simulink model "F303RE_I2S_Test"  (R2018b)
settings: Solver=FixedStepDiscrete  StartTime=0.0  StopTime=10.0  FixedStep=0.01  RelTol=1e-3
libraries: I2S_Lib x11, GPIO_Lib x7, SPI_Lib x2, DAC_Lib x1, STM32_Config_Lib x1, TIMERS_Lib x1
settings Model: Creator=reynaudp  LastModifiedBy=fenard1
settings DataIOCC: ReturnWorkspaceOutputs=on
settings OptimizationCC: DefaultParameterBehavior=Inlined  DefaultUnderspecifiedDataType=single
settings DebuggingCC: ReadBeforeWriteMsg=DisableAll  WriteAfterWriteMsg=DisableAll  WriteAfterReadMsg=DisableAll  MultiTaskDSMMsg=none  ParameterTunabilityLossMsg=error  SFUndirectedBroadcastEventsDiag=error
settings HardwareCC: ProdBitPerPointer=32  ProdBitPerSizeT=32  ProdBitPerPtrDiffT=32  ProdLargestAtomicInteger=Integer  ProdWordSize=32  ProdHWDeviceType=STMicroelectronics->STM32 32-bit Cortex-M
settings ModelReferenceCC: UpdateModelReferenceTargets=IfOutOfDate
settings SFSimCC: SFSimEcho=off  SimUseLocalCustomCode=off  CompileTimeRecursionLimit=0  EnableRuntimeRecursion=off  MATLABDynamicMemAlloc=off
settings RTWCC: SystemTargetFile=stm32.tlc  TemplateMakefile=stm32.tmf  Description=stm32 (Embedded Target)  GenerateReport=on  RTWUseLocalCustomCode=off  IncludeHyperlinkInReport=on
settings CodeAppCC: ForceParamTrailComments=on  IgnoreCustomStorageClasses=off  OperatorAnnotations=on  SimulinkDataObjDesc=on  SFDataObjDesc=on  MATLABFcnDesc=on  CustomSymbolStrType=$N$R$M  SimulinkBlockComments=off  MATLABSourceComments=on
settings STFCustomTargetCC: TargetLangStandard=C99 (ISO)  ParMdlRefBuildCompliant=on  IncludeMdlTerminateFcn=off  CombineOutputUpdateFcns=on  ERTCustomFileBanners=on  SupportNonFinite=off  SupportComplex=off  SupportContinuousTime=off  SupportNonInlinedSFcns=off  RemoveResetFunc=on  ParenthesesLevel=Maximum  CastingMode=Standards  MATLABClassNameForMDSCustomization=Simulink.SoftwareTarget.ERTCustomization  SystemTargetFile=stm32.tlc
settings ERTTargetCC: TargetLangStandard=C99 (ISO)  MultiwordLength=2048  CompOptLevelCompliant=off  ConcurrentExecutionCompliant=off  IncludeMdlTerminateFcn=off  SupportNonFinite=off  SupportComplex=off  ParenthesesLevel=Maximum  CastingMode=Standards  ModelStepFunctionPrototypeControlCompliant=off  CPPClassGenCompliant=off  UseToolchainInfoCompliant=off  ExtModeStaticAllocSize=256  ExtModeMexArgs=0,1,115200,10  InlinedParameterPlacement=NonHierarchical  ERTSrcFileBannerTemplate=sourceFileTemplate.cgt  ERTHdrFileBannerTemplate=sourceFileTemplate.cgt  ERTDataSrcFileTemplate=sourceFileTemplate.cgt  ERTDataHdrFileTemplate=sourceFileTemplate.cgt  ERTCustomFileTemplate=customRoutineProcess.tlc  PreserveIfCondition=on  EnableSignedLeftShifts=off  EnableSignedRightShifts=off

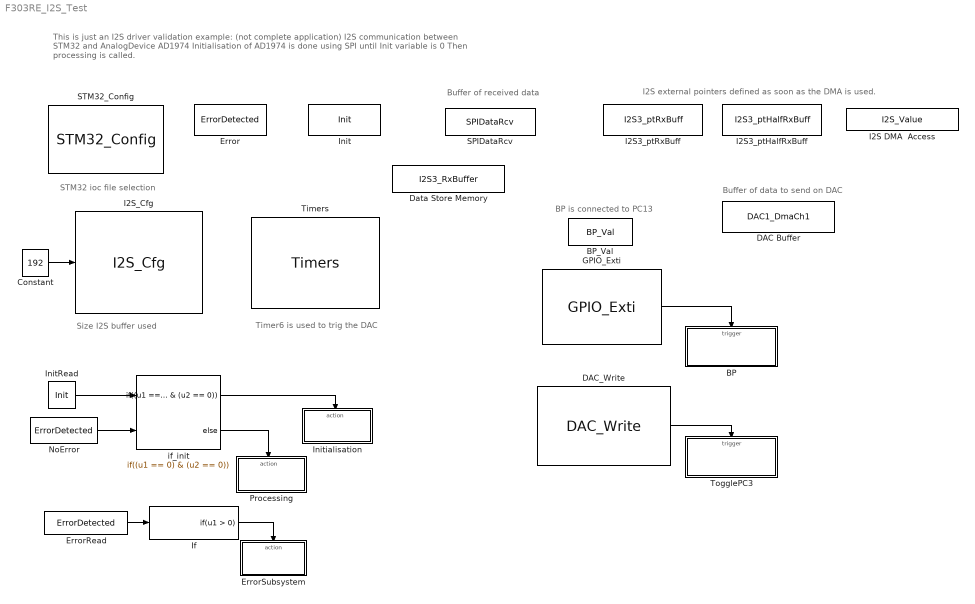
== system F303RE_I2S_Test ==
  note: Size I2S buffer used
  note: Timer6 is used to trig the DAC
  note: BP is connected to PC13
  note: Buffer of data to send on DAC
  note: Buffer of received data
  note: I2S external pointers defined as soon as the DMA is used.
  note: This is just an I2S driver validation example: (not complete application)
      | I2S communication between STM32 and AnalogDevice AD1974
      | Initialisation of AD1974 is done using SPI until Init variable is 0
      | Then processing is called.
  note: STM32 ioc file selection
  BP : Subsystem  TreatAsAtomicUnit=on
  BP_Val : DataStoreMemory  DataStoreName=BP_Val  ReadBeforeWriteMsg=warning  WriteAfterWriteMsg=warning  WriteAfterReadMsg=warning  InitialValue=1  ShowAdditionalParam=off  OutDataTypeStr=uint8
  Constant : Constant  Value=192  OutDataTypeStr=uint8
  DAC Buffer : DataStoreMemory  DataStoreName=DAC1_DmaCh1  ReadBeforeWriteMsg=warning  WriteAfterWriteMsg=warning  WriteAfterReadMsg=warning  ShowAdditionalParam=off  OutDataTypeStr=uint16  Dimensions=48
      settings: RTWStateStorageClass=ImportedExternPointer
  DAC_Write : DAC_Lib/DAC_Write  DAC_Name=DAC1  Pin0=off  Pin1=off  Align=12bit_right  DmaBuffCh1=48  DmaBuffCh2=0  CpltTrans=on  HalfTrans=off  ErrorIt=off  UnderIt=off  NbDAC=1  UsedDma=on
      settings: SourceProductName=Target Support Package - STM32 Adapter
  Data Store Memory : DataStoreMemory  DataStoreName=I2S3_RxBuffer  ReadBeforeWriteMsg=warning  WriteAfterWriteMsg=warning  WriteAfterReadMsg=warning  ShowAdditionalParam=off  Dimensions=192
  Error : DataStoreMemory  DataStoreName=ErrorDetected  ReadBeforeWriteMsg=warning  WriteAfterWriteMsg=warning  WriteAfterReadMsg=warning  ShowAdditionalParam=off  OutDataTypeStr=uint8
  ErrorRead : DataStoreRead  DataStoreName=ErrorDetected
  ErrorSubsystem : Subsystem  TreatAsAtomicUnit=on
  GPIO_Exti : GPIO_Lib/GPIO_Exti  Port_name=GPIOC  Pin_0=off  Pin_1=off  Pin_2=off  Pin_3=off  Pin_4=off  Pin_5=off  Pin_6=off  Pin_7=off  Pin_8=off  Pin_9=off  Pin_10=off  Pin_11=off  Pin_12=off  Pin_13=on  Pin_14=off  Pin_15=off  PinList=GPIOA9GPIOC13
      settings: SourceProductName=Target Support Package - STM32 Adapter
  I2S DMA  Access : DataStoreMemory  DataStoreName=I2S_Value  ReadBeforeWriteMsg=warning  WriteAfterWriteMsg=warning  WriteAfterReadMsg=warning  ShowAdditionalParam=off  OutDataTypeStr=uint16  Dimensions=96
  I2S3_ptHalfRxBuff : DataStoreMemory  DataStoreName=I2S3_ptHalfRxBuff  ReadBeforeWriteMsg=warning  WriteAfterWriteMsg=warning  WriteAfterReadMsg=warning  ShowAdditionalParam=off  OutDataTypeStr=uint16  Dimensions=96
      settings: RTWStateStorageClass=ImportedExternPointer
  I2S3_ptRxBuff : DataStoreMemory  DataStoreName=I2S3_ptRxBuff  ReadBeforeWriteMsg=warning  WriteAfterWriteMsg=warning  WriteAfterReadMsg=warning  ShowAdditionalParam=off  OutDataTypeStr=uint16  Dimensions=96
      settings: RTWStateStorageClass=ImportedExternPointer
  I2S_Cfg : I2S_Lib/I2S_Cfg  I2Sx=I2S3  Master_Slave=MASTER  Half_Full=HALF DUPLEX  Rx_Tx=Receiver  I2S_Mode=DMA_RX  NbI2S=1  Rx_SizeIn=off  Rx_Size=192  Tx_SizeIn=on  Tx_Size=192
      settings: SourceProductName=Target Support Package - STM32 Adapter  DataFormat=16 Bits Data on 32 Bits Frame
  If : If  ShowElse=off
  Init : DataStoreMemory  DataStoreName=Init  ReadBeforeWriteMsg=warning  WriteAfterWriteMsg=warning  WriteAfterReadMsg=warning  ShowAdditionalParam=off  OutDataTypeStr=uint8
  InitRead : DataStoreRead  DataStoreName=Init
  Initialisation : Subsystem  TreatAsAtomicUnit=on
  NoError : DataStoreRead  DataStoreName=ErrorDetected
  Processing : Subsystem  TreatAsAtomicUnit=on
  SPIDataRcv : DataStoreMemory  DataStoreName=SPIDataRcv  ReadBeforeWriteMsg=warning  WriteAfterWriteMsg=warning  WriteAfterReadMsg=warning  ShowAdditionalParam=off  OutDataTypeStr=uint8  Dimensions=3
  STM32_Config : STM32_Config_Lib/STM32_Config  Priority=0  Project_Path=.\  Config_File=F303RE.ioc  MCU_Name=STM32F303RETx
      settings: SourceProductName=Target Support Package - STM32 Adapter
  Timers : TIMERS_Lib/Timers  currentTIM=TIM6  TIM_Name=TIM6  sysUsingTimer=on  TIM_APBClock=72000000  TIM_Set_Clk=off  TIM_Prescaler=9  TIM_Clock=7200000.00  Variable_frequency=off  TIM_Set_OutFreq=on  TIM_ARR=150  Output_frequency=48000.00  Repetition_counter=0  TIM_Mode=Up  TIM_DMA=none  TIM_IRQ=off  TIM_IRQ_ONLY=on  TIM_UP=off  TIM_TRG=off  TIM_COM=off  TIM_BRK=off  NbTIM=1  CH1_enable=off  CH1N_enable=off  CH1_type=Unknown  CH1_DMA=off  CH1_int=off  CH1_edge=Rising  CH1_div=1  CH1_variable_duty=off  CH1_set_pulse=off  CH1_output_duty=0.00  CH1_pulse=0  CH2_enable=off  CH2N_enable=off  CH2_type=Unknown  CH2_DMA=off  CH2_int=off  CH2_edge=Rising  CH2_div=1  CH2_variable_duty=off  CH2_set_pulse=off  CH2_output_duty=0.00  CH2_pulse=0  CH3_enable=off  CH3N_enable=off  CH3_type=Unknown  CH3_DMA=off  CH3_int=off  CH3_edge=Rising  CH3_div=1  CH3_variable_duty=off  CH3_set_pulse=off  CH3_output_duty=0.00  CH3_pulse=0  CH4_enable=off  CH4N_enable=off  CH4_type=Unknown  CH4_DMA=off  CH4_int=off  CH4_edge=Rising  CH4_div=1  CH4_variable_duty=off  CH4_set_pulse=off  CH4_output_duty=0.00  CH4_pulse=0
      settings: SourceProductName=Target Support Package - STM32 Adapter
  TogglePC3 : Subsystem  TreatAsAtomicUnit=on
  if_init : If  NumInputs=2  IfExpression=(u1 == 0) & (u2 == 0)
  wires:
  ErrorRead/1 -> If/1
  If/1 -> ErrorSubsystem/Action
  InitRead/1 -> if_init/1
  NoError/1 -> if_init/2
  if_init/1 -> Initialisation/Action
  if_init/2 -> Processing/Action
  DAC_Write/1 -> TogglePC3/Trigger
  GPIO_Exti/1 -> BP/Trigger
  Constant/1 -> I2S_Cfg/1

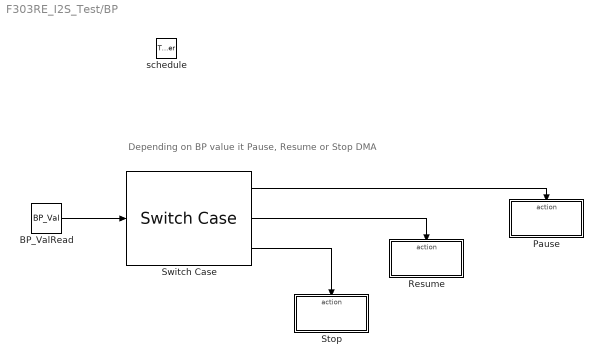
== system F303RE_I2S_Test/BP ==
  note: Depending on BP value it Pause, Resume or Stop DMA
  schedule : TriggerPort  TriggerType=function-call  VariantControl=Variant
  BP_ValRead : DataStoreRead  DataStoreName=BP_Val
  Pause : Subsystem  TreatAsAtomicUnit=on
  Resume : Subsystem  TreatAsAtomicUnit=on
  Stop : Subsystem  TreatAsAtomicUnit=on
  Switch Case : SwitchCase  CaseConditions={1,2,3}  ShowDefaultCase=off
  wires:
  BP_ValRead/1 -> Switch Case/1
  Switch Case/1 -> Pause/Action
  Switch Case/2 -> Resume/Action
  Switch Case/3 -> Stop/Action

== system F303RE_I2S_Test/ErrorSubsystem ==
  note: Blink LED
  Action Port : ActionPort  ActionType=then
  GPIO_Write : GPIO_Lib/GPIO_Write  Port_name=GPIOB  Pin0=off  Toggle_Pin0=off  Pin1=off  Toggle_Pin1=off  Pin2=off  Toggle_Pin2=off  Pin3=off  Toggle_Pin3=off  Pin4=off  Toggle_Pin4=off  Pin5=off  Toggle_Pin5=off  Pin6=off  Toggle_Pin6=off  Pin7=off  Toggle_Pin7=off  Pin8=off  Toggle_Pin8=off  Pin9=off  Toggle_Pin9=off  Pin10=off  Toggle_Pin10=off  Pin11=off  Toggle_Pin11=off  Pin12=off  Toggle_Pin12=off  Pin13=off  Toggle_Pin13=off  Pin14=off  Toggle_Pin14=off  Pin15=off  Toggle_Pin15=off  PinList="GPIOA8  10GPIOB3  6GPIOC3"
      settings: SourceProductName=Target Support Package - STM32 Adapter

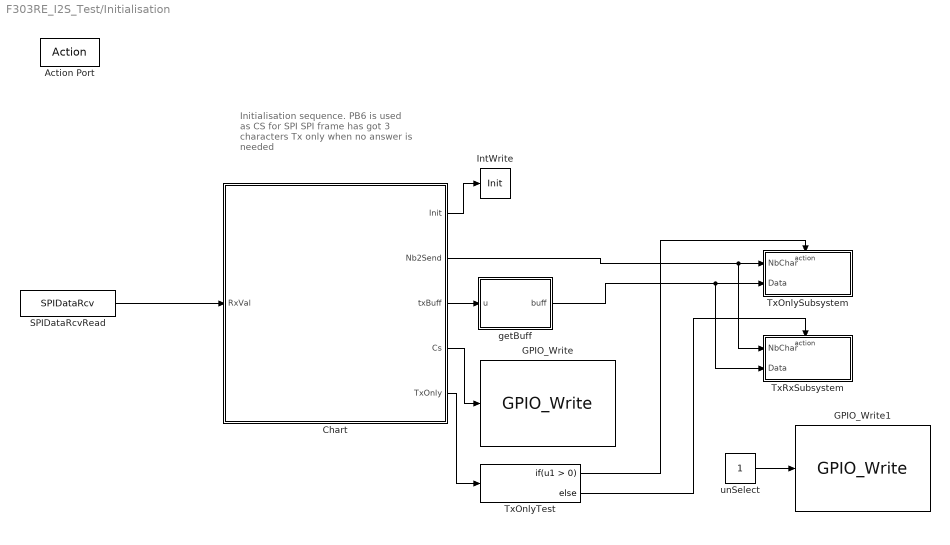
== system F303RE_I2S_Test/Initialisation ==
  note: Initialisation sequence.
      | PB6 is used as CS for SPI
      | SPI frame has got 3 characters
      | Tx only when no answer is needed
  Action Port : ActionPort  ActionType=then
  Chart : Stateflow chart  TreatAsAtomicUnit=on
  GPIO_Write : GPIO_Lib/GPIO_Write  Priority=0  Port_name=GPIOB  Pin0=off  Toggle_Pin0=off  Pin1=off  Toggle_Pin1=off  Pin2=off  Toggle_Pin2=off  Pin3=off  Toggle_Pin3=off  Pin4=off  Toggle_Pin4=off  Pin5=off  Toggle_Pin5=off  Pin6=on  Toggle_Pin6=off  Pin7=off  Toggle_Pin7=off  Pin8=off  Toggle_Pin8=off  Pin9=off  Toggle_Pin9=off  Pin10=off  Toggle_Pin10=off  Pin11=off  Toggle_Pin11=off  Pin12=off  Toggle_Pin12=off  Pin13=off  Toggle_Pin13=off  Pin14=off  Toggle_Pin14=off  Pin15=off  Toggle_Pin15=off  PinList="GPIOA8  10GPIOB3  6GPIOC3"
      settings: SourceProductName=Target Support Package - STM32 Adapter
  GPIO_Write1 : GPIO_Lib/GPIO_Write  Priority=2  Port_name=GPIOB  Pin0=off  Toggle_Pin0=off  Pin1=off  Toggle_Pin1=off  Pin2=off  Toggle_Pin2=off  Pin3=off  Toggle_Pin3=off  Pin4=off  Toggle_Pin4=off  Pin5=off  Toggle_Pin5=off  Pin6=on  Toggle_Pin6=off  Pin7=off  Toggle_Pin7=off  Pin8=off  Toggle_Pin8=off  Pin9=off  Toggle_Pin9=off  Pin10=off  Toggle_Pin10=off  Pin11=off  Toggle_Pin11=off  Pin12=off  Toggle_Pin12=off  Pin13=off  Toggle_Pin13=off  Pin14=off  Toggle_Pin14=off  Pin15=off  Toggle_Pin15=off  PinList="GPIOA8  10GPIOB3  6GPIOC3"
      settings: SourceProductName=Target Support Package - STM32 Adapter
  IntWrite : DataStoreWrite  DataStoreName=Init
  SPIDataRcvRead : DataStoreRead  DataStoreName=SPIDataRcv
  TxOnlySubsystem : Subsystem  TreatAsAtomicUnit=on
  TxOnlyTest : If
  TxRxSubsystem : Subsystem  TreatAsAtomicUnit=on
  getBuff : MATLAB Function  TreatAsAtomicUnit=on
  unSelect : Constant
  wires:
  Chart/1(Init) -> IntWrite/1
  Chart/3(txBuff) -> getBuff/1(u)
  Chart/4(Cs) -> GPIO_Write/1
  unSelect/1 -> GPIO_Write1/1
  Chart/5(TxOnly) -> TxOnlyTest/1
  TxOnlyTest/1 -> TxOnlySubsystem/Action
  TxOnlyTest/2 -> TxRxSubsystem/Action
  Chart/2(Nb2Send) -> TxRxSubsystem/1(NbChar), TxOnlySubsystem/1(NbChar)
  getBuff/1(buff) -> TxRxSubsystem/2(Data), TxOnlySubsystem/2(Data)
  SPIDataRcvRead/1 -> Chart/1(RxVal)

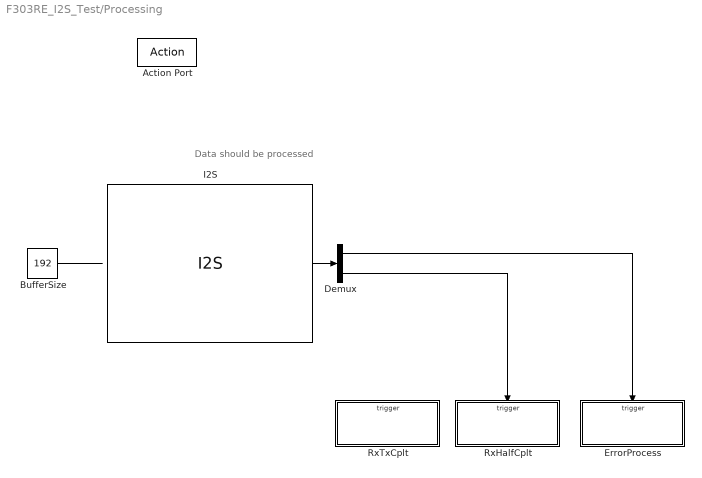
== system F303RE_I2S_Test/Processing ==
  note: Data should be processed
  Action Port : ActionPort  ActionType=else
  BufferSize : Constant  Value=192
  Demux : Demux  Outputs=2
  ErrorProcess : Subsystem  TreatAsAtomicUnit=on
  I2S : I2S_Lib/I2S  I2Sx=I2S3  Master_Slave=MASTER  Half_Full=HALF DUPLEX  Rx_Tx=Receiver  ptDataSent=off  Protocol=I2S Philips  Frequency=48 KHz  RealFrequency=46.875 KHz  FrequencyError=-2.34 %  ClockPol=Low  I2S_Mode=DMA_RX  Timeout=-1  TimeoutValue=0.01  handler=hi2s3  NbI2S=1  Error=on  RxHalfCplt=on  RxCplt=off  TxHalfCplt=off  TxCplt=off  RxTxCplt=off  outputData=off
      settings: SourceProductName=Target Support Package - STM32 Adapter  DataFormat=16 Bits Data on 32 Bits Frame
  RxHalfCplt : Subsystem  TreatAsAtomicUnit=on
  RxTxCplt : Subsystem  TreatAsAtomicUnit=on
  wires:
  BufferSize/1 -> ?
  I2S/1 -> Demux/1
  Demux/1 -> ErrorProcess/Trigger
  Demux/2 -> RxHalfCplt/Trigger

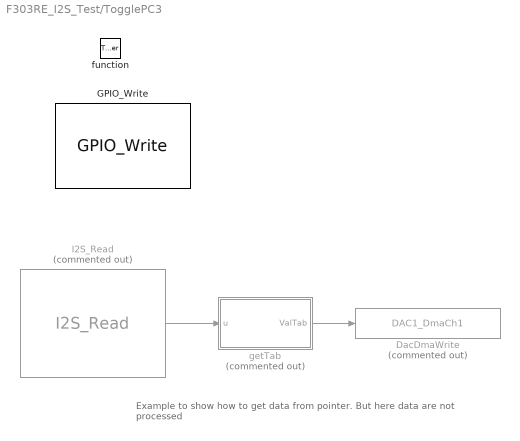
== system F303RE_I2S_Test/TogglePC3 ==
  note: Example to show how to get data from pointer.
      |
      | But here data are not processed
  function : TriggerPort  TriggerType=function-call  VariantControl=Variant
  DacDmaWrite : DataStoreWrite  Commented=on  DataStoreName=DAC1_DmaCh1
  GPIO_Write : GPIO_Lib/GPIO_Write  Port_name=GPIOB  Pin0=off  Toggle_Pin0=off  Pin1=off  Toggle_Pin1=off  Pin2=off  Toggle_Pin2=off  Pin3=off  Toggle_Pin3=off  Pin4=off  Toggle_Pin4=off  Pin5=off  Toggle_Pin5=off  Pin6=off  Toggle_Pin6=off  Pin7=off  Toggle_Pin7=off  Pin8=off  Toggle_Pin8=off  Pin9=off  Toggle_Pin9=off  Pin10=off  Toggle_Pin10=off  Pin11=off  Toggle_Pin11=off  Pin12=off  Toggle_Pin12=off  Pin13=off  Toggle_Pin13=off  Pin14=off  Toggle_Pin14=off  Pin15=off  Toggle_Pin15=off  PinList="GPIOA8  10GPIOB3  6GPIOC3"
      settings: SourceProductName=Target Support Package - STM32 Adapter
  I2S_Read : I2S_Lib/I2S_Read  Commented=on  I2Sx=I2S3  OffsetIn=off  OffsetVal=0  outputData=on
      settings: SourceProductName=Target Support Package - STM32 Adapter
  getTab : MATLAB Function  Commented=on  TreatAsAtomicUnit=on
  wires:
  I2S_Read/2 -> getTab/1(u)
  getTab/1(ValTab) -> DacDmaWrite/1

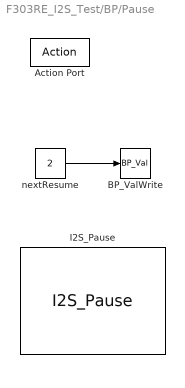
== system F303RE_I2S_Test/BP/Pause ==
  Action Port : ActionPort  ActionType=case
  BP_ValWrite : DataStoreWrite  DataStoreName=BP_Val
  I2S_Pause : I2S_Lib/I2S_Pause  I2Sx=I2S3
      settings: SourceProductName=Target Support Package - STM32 Adapter
  nextResume : Constant  Value=2  OutDataTypeStr=uint8
  wires:
  nextResume/1 -> BP_ValWrite/1

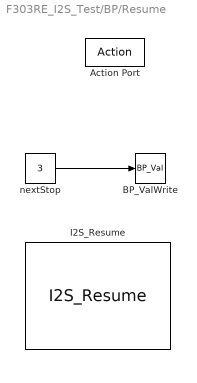
== system F303RE_I2S_Test/BP/Resume ==
  Action Port : ActionPort  ActionType=case
  BP_ValWrite : DataStoreWrite  DataStoreName=BP_Val
  I2S_Resume : I2S_Lib/I2S_Resume  I2Sx=I2S3
      settings: SourceProductName=Target Support Package - STM32 Adapter
  "nextStop " : Constant  Value=3  OutDataTypeStr=uint8
  wires:
  "nextStop "/1 -> BP_ValWrite/1

== system F303RE_I2S_Test/BP/Stop ==
  Action Port : ActionPort  ActionType=case
  BP_ValWrite : DataStoreWrite  DataStoreName=BP_Val
  I2S_Stop : I2S_Lib/I2S_Stop  I2Sx=I2S3
      settings: SourceProductName=Target Support Package - STM32 Adapter
  nextEnd : Constant  Value=0  OutDataTypeStr=uint8
  wires:
  nextEnd/1 -> BP_ValWrite/1

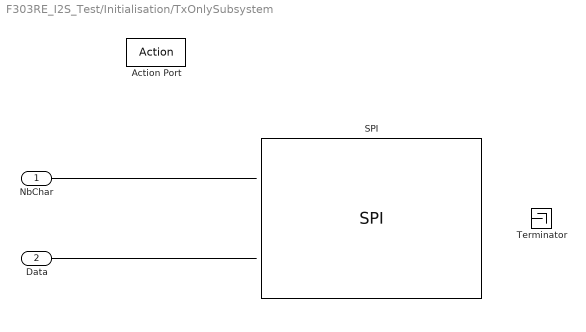
== system F303RE_I2S_Test/Initialisation/TxOnlySubsystem ==
  NbChar : Inport
  Data : Inport  Port=2
  Action Port : ActionPort  ActionType=then
  SPI : SPI_Lib/SPI  SPIx=SPI1  Device_Mode=MASTER  Type_SPI=Full_Duplex  SPI_Mode=POLLING  TxOnly=on  handler=hspi1  Buffer_Size_Rcv=32  Buffer_Size_Send=32  NbSPI=1  BaudRate=1.125 MBits/s  Nb_bits_transmission=8  Timeout=200  TimeoutValue=2  NSS=off  Error=off  CallBack=off  Transmission=off  outputData=off
      settings: SourceProductName=Target Support Package - STM32 Adapter
  Terminator : Terminator
  wires:
  NbChar/1 -> ?
  Data/1 -> ?
  ? -> Terminator/1

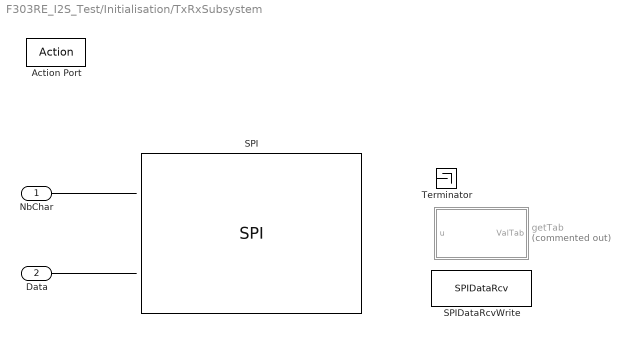
== system F303RE_I2S_Test/Initialisation/TxRxSubsystem ==
  NbChar : Inport
  Data : Inport  Port=2
  Action Port : ActionPort  ActionType=else
  SPI : SPI_Lib/SPI  Priority=1  SPIx=SPI1  Device_Mode=MASTER  Type_SPI=Full_Duplex  SPI_Mode=POLLING  TxOnly=off  handler=hspi1  Buffer_Size_Rcv=3  Buffer_Size_Send=3  NbSPI=1  BaudRate=1.125 MBits/s  Nb_bits_transmission=8  Timeout=200  TimeoutValue=2  NSS=off  Error=off  CallBack=off  Transmission=off  outputData=on
      settings: SourceProductName=Target Support Package - STM32 Adapter
  SPIDataRcvWrite : DataStoreWrite  DataStoreName=SPIDataRcv
  Terminator : Terminator
  getTab : MATLAB Function  Commented=on  TreatAsAtomicUnit=on
  wires:
  NbChar/1 -> ?
  Data/1 -> ?
  ? -> SPIDataRcvWrite/1
  ? -> getTab/1(u)
  ? -> Terminator/1

== system F303RE_I2S_Test/Processing/ErrorProcess ==
  ProcessError : TriggerPort  TriggerType=function-call  VariantControl=Variant
  Constant : Constant  OutDataTypeStr=uint8
  ErrorWrite : DataStoreWrite  DataStoreName=ErrorDetected
  wires:
  Constant/1 -> ErrorWrite/1

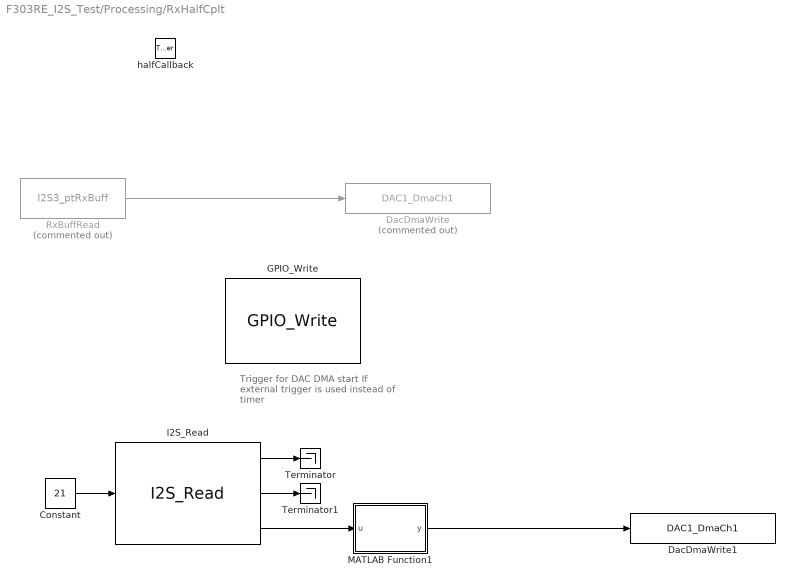
== system F303RE_I2S_Test/Processing/RxHalfCplt ==
  note: Trigger for DAC DMA start
      | If external trigger is used instead of timer
  halfCallback : TriggerPort  TriggerType=function-call  VariantControl=Variant
  Constant : Constant  Value=21  OutDataTypeStr=uint16
  DacDmaWrite : DataStoreWrite  Commented=on  DataStoreName=DAC1_DmaCh1
  DacDmaWrite1 : DataStoreWrite  DataStoreName=DAC1_DmaCh1
  GPIO_Write : GPIO_Lib/GPIO_Write  Port_name=GPIOB  Pin0=off  Toggle_Pin0=off  Pin1=off  Toggle_Pin1=off  Pin2=off  Toggle_Pin2=off  Pin3=off  Toggle_Pin3=off  Pin4=off  Toggle_Pin4=off  Pin5=off  Toggle_Pin5=off  Pin6=off  Toggle_Pin6=off  Pin7=off  Toggle_Pin7=off  Pin8=off  Toggle_Pin8=off  Pin9=off  Toggle_Pin9=off  Pin10=off  Toggle_Pin10=off  Pin11=off  Toggle_Pin11=off  Pin12=off  Toggle_Pin12=off  Pin13=off  Toggle_Pin13=off  Pin14=off  Toggle_Pin14=off  Pin15=off  Toggle_Pin15=off  PinList="GPIOA8  10GPIOB3  6GPIOC3"
      settings: SourceProductName=Target Support Package - STM32 Adapter
  I2S_Read : I2S_Lib/I2S_Read  I2Sx=I2S3  OffsetIn=on  OffsetVal=0  outputData=on
      settings: SourceProductName=Target Support Package - STM32 Adapter
  MATLAB Function1 : MATLAB Function  TreatAsAtomicUnit=on
  RxBuffRead : DataStoreRead  Commented=on  DataStoreName=I2S3_ptRxBuff
  Terminator : Terminator
  Terminator1 : Terminator
  wires:
  RxBuffRead/1 -> DacDmaWrite/1
  I2S_Read/3 -> MATLAB Function1/1(u)
  MATLAB Function1/1(y) -> DacDmaWrite1/1
  Constant/1 -> I2S_Read/1
  I2S_Read/1 -> Terminator/1
  I2S_Read/2 -> Terminator1/1

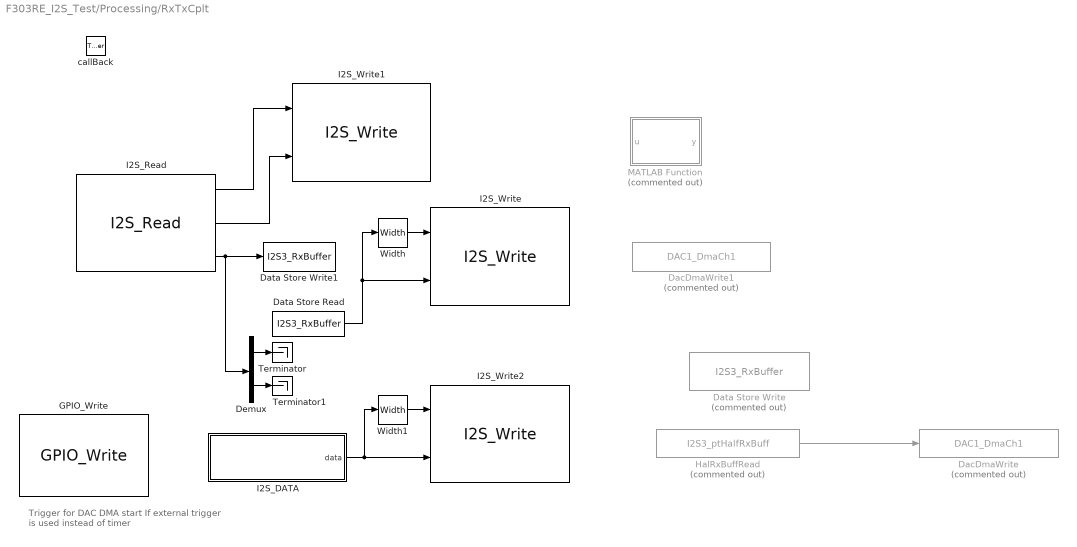
== system F303RE_I2S_Test/Processing/RxTxCplt ==
  note: Trigger for DAC DMA start
      | If external trigger is used instead of timer
  callBack : TriggerPort  TriggerType=function-call  VariantControl=Variant
  DacDmaWrite : DataStoreWrite  Commented=on  DataStoreName=DAC1_DmaCh1
  DacDmaWrite1 : DataStoreWrite  Commented=on  DataStoreName=DAC1_DmaCh1
  Data Store Read : DataStoreRead  DataStoreName=I2S3_RxBuffer
  Data Store Write : DataStoreWrite  Commented=on  DataStoreName=I2S3_RxBuffer
  Data Store Write1 : DataStoreWrite  DataStoreName=I2S3_RxBuffer
  Demux : Demux  Outputs=2
  GPIO_Write : GPIO_Lib/GPIO_Write  Port_name=GPIOB  Pin0=off  Toggle_Pin0=off  Pin1=off  Toggle_Pin1=off  Pin2=off  Toggle_Pin2=off  Pin3=off  Toggle_Pin3=off  Pin4=off  Toggle_Pin4=off  Pin5=off  Toggle_Pin5=off  Pin6=off  Toggle_Pin6=off  Pin7=off  Toggle_Pin7=off  Pin8=off  Toggle_Pin8=off  Pin9=off  Toggle_Pin9=off  Pin10=off  Toggle_Pin10=off  Pin11=off  Toggle_Pin11=off  Pin12=off  Toggle_Pin12=off  Pin13=off  Toggle_Pin13=off  Pin14=off  Toggle_Pin14=off  Pin15=off  Toggle_Pin15=off  PinList="GPIOA8  10GPIOB3  6GPIOC3"
      settings: SourceProductName=Target Support Package - STM32 Adapter
  HalRxBuffRead : DataStoreRead  Commented=on  DataStoreName=I2S3_ptHalfRxBuff
  I2S_DATA : Subsystem
  I2S_Read : I2S_Lib/I2S_Read  I2Sx=I2S3  OffsetIn=off  OffsetVal=3  outputData=on
      settings: SourceProductName=Target Support Package - STM32 Adapter
  I2S_Write : I2S_Lib/I2S_Write  I2Sx=I2S3  inputData=on  dataMsg=BufferDataSend is the data to copy to the send buffer  OffsetIn=off  OffsetVal=12
      settings: SourceProductName=Target Support Package - STM32 Adapter  DataFormat=16 Bits Data on 32 Bits Frame
  I2S_Write1 : I2S_Lib/I2S_Write  I2Sx=I2S3  inputData=off  dataMsg=ptDataSend is the address of the data to copy to the send buffer  OffsetIn=off  OffsetVal=50
      settings: SourceProductName=Target Support Package - STM32 Adapter  DataFormat=16 Bits Data on 32 Bits Frame
  I2S_Write2 : I2S_Lib/I2S_Write  I2Sx=I2S3  inputData=on  dataMsg=BufferDataSend is the data to copy to the send buffer  OffsetIn=off  OffsetVal=12
      settings: SourceProductName=Target Support Package - STM32 Adapter  DataFormat=16 Bits Data on 32 Bits Frame
  MATLAB Function : MATLAB Function  Commented=on  TreatAsAtomicUnit=on
  Terminator : Terminator
  Terminator1 : Terminator
  Width : Width
  Width1 : Width
  wires:
  HalRxBuffRead/1 -> DacDmaWrite/1
  I2S_Read/3 -> Demux/1, Data Store Write1/1
  I2S_Read/1 -> I2S_Write1/1
  I2S_Read/2 -> I2S_Write1/2
  Data Store Read/1 -> Width/1, I2S_Write/2
  Width/1 -> I2S_Write/1
  I2S_DATA/1(data) -> Width1/1, I2S_Write2/2
  Width1/1 -> I2S_Write2/1
  Demux/1 -> Terminator/1
  Demux/2 -> Terminator1/1

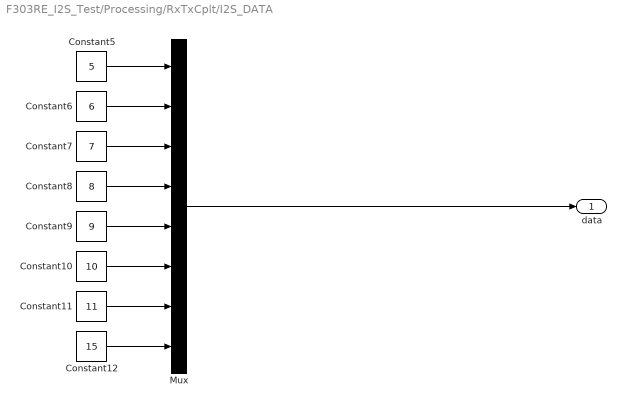
== system F303RE_I2S_Test/Processing/RxTxCplt/I2S_DATA ==
  Constant10 : Constant  Value=10  OutDataTypeStr=uint8
  Constant11 : Constant  Value=11  OutDataTypeStr=uint8
  Constant12 : Constant  Value=15  OutDataTypeStr=uint8
  Constant5 : Constant  Value=5  OutDataTypeStr=uint8
  Constant6 : Constant  Value=6  OutDataTypeStr=uint8
  Constant7 : Constant  Value=7  OutDataTypeStr=uint8
  Constant8 : Constant  Value=8  OutDataTypeStr=uint8
  Constant9 : Constant  Value=9  OutDataTypeStr=uint8
  Mux : Mux  Inputs=8
  data : Outport
  wires:
  Mux/1 -> data/1
  Constant5/1 -> Mux/1
  Constant6/1 -> Mux/2
  Constant9/1 -> Mux/5
  Constant10/1 -> Mux/6
  Constant7/1 -> Mux/3
  Constant12/1 -> Mux/8
  Constant8/1 -> Mux/4
  Constant11/1 -> Mux/7

== matlab function F303RE_I2S_Test/Initialisation/getBuff ==
  data: u input; buff output uint32 size=1
function buff = getBuff(u)
if coder.target('Sfun')
    % Executing in MATLAB, Buff is null
    buff = uint32(0);
else
    coder.cinclude('getBuffPtr.h');
    % Executing in the generated code.
    %buffer = zeros(1,3,'uint8');
    %coder.ceval('memcpy',coder.wref(buffer),coder.rref(u),3);
    %y = uint8(buffer(1:3));
    %buff = uint32(coder.ref(y));
    buff = coder.ceval('getBuffPtr',coder.rref(u));
end
end

== matlab function F303RE_I2S_Test/TogglePC3/getTab ==
  data: u input; ValTab output
function ValTab = I2SToDAC(u)
if coder.target('Sfun')
% Executing in MATLAB, Buff is null
ValTab = zeros(1,48,'uint8');
else
% Executing in the generated code. 
% Twist coder functions in order  to use input as a pointer.
ValTab = zeros(1,48,'uint8');
ptI2SData = coder.opaque('unsigned short*','0');
coder.ceval('ptI2SData=(unsigned short*)',u);
coder.ceval('memcpy',coder.wref(ValTab),ptI2SData,48);
end
end

== stateflow chart F303RE_I2S_Test/Initialisation/Chart ==
  state DumyRead
    en:
    txBuff[0] = uint8(9);
    txBuff[1] = uint8(0);
    txBuff[2] = uint8(0);
    ex: Nb2Send = uint8(3);
    Init = uint8(0);
    Cs = uint8(0);
    TxOnly = uint8(0);
  state DumyRead2
    entry: txBuff[0] = uint8(9);
    txBuff[1] = uint8(0);
    txBuff[2] = uint8(0);
    Nb2Send = uint8(3);
    Init = uint8(0);
    Cs = uint8(0);
    TxOnly = uint8(0);
  state DumyRead4
    entry: txBuff[0] = uint8(9);
    txBuff[1] = uint8(0);
    txBuff[2] = uint8(0);
    Nb2Send = uint8(3);
    Init = uint8(0);
    Cs = uint8(0);
    TxOnly = uint8(0);
  state WORDLENGTH_16
    entry: txBuff[0] = uint8(8);
    txBuff[1] = uint8(15);
    txBuff[2] = uint8(3);
    Nb2Send = uint8(3);
    Init = uint8(0);
    Cs = uint8(0);
    TxOnly = uint8(1);
  state PLL_OFF
    entry: txBuff[0] = uint8(8);
    txBuff[1] = uint8(0);
    txBuff[2] = uint8(1);
    Nb2Send = uint8(3);
    Init = uint8(0);
    Cs = uint8(0);
    TxOnly = uint8(1);
  state PLL_LOCK
    entry: txBuff[0] = uint8(9);
    txBuff[1] = uint8(1);
    txBuff[2] = uint8(0);
    Nb2Send = uint8(3);
    Init = uint8(0);
    Cs = uint8(0);
    TxOnly = uint8(0);
  state WORDLENGTH_Read
    entry: txBuff[0] = uint8(9);
    txBuff[1] = uint8(15);
    txBuff[2] = uint8(3);
    Nb2Send = uint8(3);
    Init = uint8(0);
    Cs = uint8(0);
    TxOnly = uint8(0);
  state DumyRead1
    entry: txBuff[0] = uint8(9);
    txBuff[1] = uint8(0);
    txBuff[2] = uint8(0);
    Nb2Send = uint8(3);
    Init = uint8(0);
    Cs = uint8(0);
    TxOnly = uint8(0);
  state HP_FILTER_ON
    entry: txBuff[0] = uint8(8);
    txBuff[1] = uint8(14);
    txBuff[2] = uint8(50);
    Nb2Send = uint8(3);
    Init = uint8(0);
    Cs = uint8(0);
    TxOnly = uint8(1);
  state ENABLE_PLL
    entry: txBuff[0] = uint8(8);
    txBuff[1] = uint8(0);
    txBuff[2] = uint8(72);
    Nb2Send = uint8(3);
    Init = uint8(0);
    Cs = uint8(0);
    TxOnly = uint8(1);
  state LRCK_IN
    entry: txBuff[0] = uint8(8);
    txBuff[1] = uint8(0);
    txBuff[2] = uint8(73);
    Nb2Send = uint8(3);
    Init = uint8(0);
    Cs = uint8(0);
    TxOnly = uint8(1);
  state DumyRead5
    entry: txBuff[0] = uint8(9);
    txBuff[1] = uint8(14);
    txBuff[2] = uint8(0);
    Nb2Send = uint8(3);
    Init = uint8(0);
    Cs = uint8(0);
    TxOnly = uint8(0);
  state START_CONERSION
    entry: txBuff[0] = uint16(8);
    txBuff[1] = uint16(0);
    txBuff[2] = uint16(200);
    Nb2Send = uint16(3);
    Init = uint8(0);
    Cs = uint8(0);
    TxOnly = uint8(1);
  state DumyRead6
    entry: txBuff[0] = uint16(9);
    txBuff[1] = uint16(0);
    txBuff[2] = uint16(0);
    Nb2Send = uint16(3);
    Init = uint8(1);
    Cs = uint8(0);
    TxOnly = uint8(0);
  (default) -> DumyRead
  LRCK_IN -> DumyRead2 : [1]
  ENABLE_PLL -> DumyRead4 : [1]
  DumyRead -> PLL_OFF : [after(0.5,sec)]
  DumyRead2 -> WORDLENGTH_16 : [RxVal[1] == 73||RxVal[2] == 73]
  DumyRead4 -> PLL_LOCK : [RxVal[1] == 72||RxVal[2] == 72]
  PLL_LOCK -> PLL_LOCK [order 1] : [RxVal[1] != 8&&RxVal[2] != 8 && after(0.5,sec)]
  WORDLENGTH_16 -> WORDLENGTH_Read : [1]
  PLL_OFF -> DumyRead1 : [1]
  PLL_LOCK -> HP_FILTER_ON [order 2] : [RxVal[1] == 8||RxVal[2] == 8]
  WORDLENGTH_Read -> ENABLE_PLL : [RxVal[1] == 3||RxVal[2] == 3]
  DumyRead1 -> LRCK_IN : [RxVal[1] == 1||RxVal[2] == 1]
  HP_FILTER_ON -> DumyRead5 : [1]
  DumyRead5 -> START_CONERSION : [RxVal[1] == 50||RxVal[2] == 50]
  START_CONERSION -> DumyRead6 : [1]
  data: Init output uint8; Nb2Send output uint16; RxVal input uint8 size=3; txBuff output uint8 size=3; Cs output uint8; TxOnly output uint8

== matlab function F303RE_I2S_Test/Initialisation/TxRxSubsystem/getTab ==
  data: u input; ValTab output
function ValTab = getElems(u)
if coder.target('Sfun')
% Executing in MATLAB, Buff is null
ValTab = zeros(1,3,'uint8');
else
% Executing in the generated code. 
% Twist coder functions in order  to use input as a pointer.
ValTab = zeros(1,3,'uint8');
pt2Data = coder.opaque('unsigned short*','0');
coder.ceval('pt2Data=(unsigned short*)',u);
coder.ceval('memcpy',coder.wref(ValTab),pt2Data,3);
end
end

== matlab function F303RE_I2S_Test/Processing/RxTxCplt/MATLAB Function ==
  data: u input; y output uint16 size=48
function y = fcn(u)
 y = uint16(1:1:48)';
 for i=1:48    
    if(u(i)>=128)
        y(i) = bitxor(u(i*2) ,255,'uint16') + 1;
    else
        y(i) = u(i*2);
    end
 end
end

== matlab function F303RE_I2S_Test/Processing/RxHalfCplt/MATLAB Function1 ==
  data: u input; y output uint16 size=48
function y = fcn(u)
 y = uint16(1:1:48)';
 for i=1:48    
    if(u(i+96)>=128)
        y(i) = bitxor(u(i*2 + 96) ,255,'uint16') + 1;
    else
        y(i) = u(i*2 + 96);
    end
 end
end
